simulink model "control_pos_6dof_conMI"  (R2023b)
settings: Solver=ode45  StartTime=0.0  StopTime=tsim  FixedStep=tstep  MaxStep=tstep
undefined symbols (not defined in the file): a0, a1, MI_Contr1, MI_Contr2, MI_Contr3, MI_Contr4, MI_Contr5, MI_Contr6, MI_motor1, MI_motor2, MI_motor3, MI_motor4, MI_motor5, MI_motor6, robot_params, sigbuilder_block, t_qeq_init, t_tr_init, tau_L, tr_ref
(part 2 of 10)

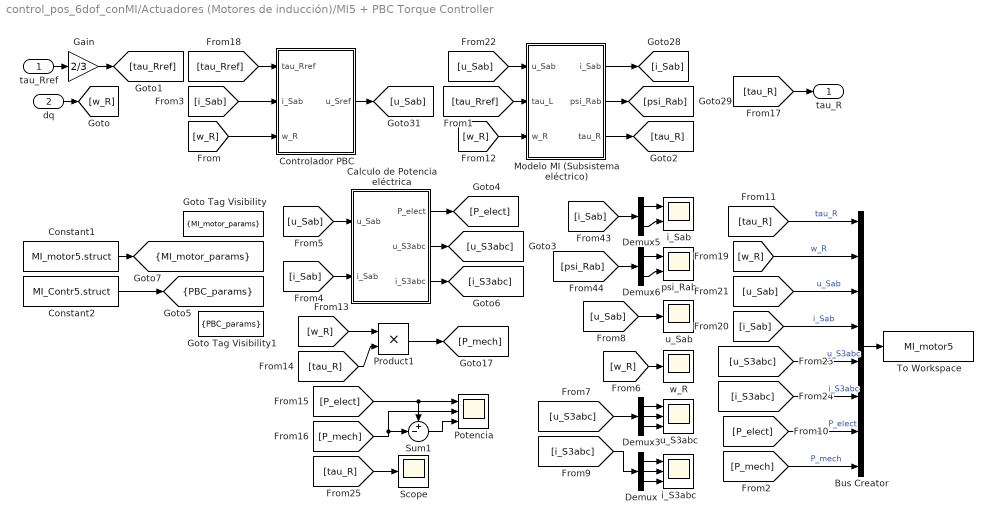
== system control_pos_6dof_conMI/Actuadores (Motores de inducción)/MI5 + PBC Torque Controller ==
  tau_Rref : Inport
  dq : Inport  Port=2
  Bus Creator : BusCreator  Inputs=8
  Calculo de Potencia eléctrica : Subsystem
  Constant1 : Constant  Value=MI_motor5.struct  OutDataTypeStr=Bus: MI_bus
  Constant2 : Constant  Value=MI_Contr5.struct  OutDataTypeStr=Bus: PBC_bus
  Controlador PBC : Subsystem
  Demux : Demux  Outputs=3
  Demux3 : Demux  Outputs=3
  Demux5 : Demux  Outputs=2
  Demux6 : Demux  Outputs=2
  Gain : Gain  Gain=2/3
  Goto Tag Visibility : GotoTagVisibility  GotoTag=MI_motor_params
  Goto Tag Visibility1 : GotoTagVisibility  GotoTag=PBC_params
  Modelo MI (Subsistema eléctrico) : Subsystem
  Potencia : Scope  NumInputPorts=3
  Product1 : Product
  Scope : Scope
  Sum1 : Sum  Inputs=+-|
  To Workspace : ToWorkspace  VariableName=MI_motor5  SaveFormat=Timeseries  SampleTime=-1
  i_S3abc : Scope  NumInputPorts=3
  i_Sab : Scope  NumInputPorts=2
  psi_Rab : Scope  NumInputPorts=2
  u_S3abc : Scope  NumInputPorts=3
  u_Sab : Scope
  w_R : Scope
  tau_R : Outport
  tag scope: MI_motor_params=scoped, PBC_params=scoped
  wires:
  Modelo MI (Subsistema eléctrico)/2(psi_Rab) -> [psi_Rab]
  [u_Sab] -> Modelo MI (Subsistema eléctrico)/1(u_Sab)
  [i_Sab] -> Controlador PBC/2(i_Sab)
  Controlador PBC/1(u_Sref) -> [u_Sab]
  [w_R] -> Controlador PBC/3(w_R)
  [tau_Rref] -> Modelo MI (Subsistema eléctrico)/2(tau_L)
  Calculo de Potencia eléctrica/2(u_S3abc) -> [u_S3abc]
  Calculo de Potencia eléctrica/1(P_elect) -> [P_elect]
  Demux5/1 -> i_Sab/1
  [w_R] -> w_R/1
  [u_Sab] -> Calculo de Potencia eléctrica/1(u_Sab)
  [psi_Rab] -> Demux6/1
  [u_Sab] -> u_Sab/1
  Demux6/1 -> psi_Rab/1
  Calculo de Potencia eléctrica/3(i_S3abc) -> [i_S3abc]
  Demux6/2 -> psi_Rab/2
  Demux5/2 -> i_Sab/2
  [i_Sab] -> Calculo de Potencia eléctrica/2(i_Sab)
  [i_Sab] -> Demux5/1
  Demux/2 -> i_S3abc/2
  Demux3/1 -> u_S3abc/1
  Demux3/3 -> u_S3abc/3
  [i_S3abc] -> Demux/1
  Demux/1 -> i_S3abc/1
  Demux/3 -> i_S3abc/3
  [u_S3abc] -> Demux3/1
  Demux3/2 -> u_S3abc/2
  Modelo MI (Subsistema eléctrico)/1(i_Sab) -> [i_Sab]
  Modelo MI (Subsistema eléctrico)/3(tau_R) -> [tau_R]
  Product1/1 -> [P_mech]
  [w_R] -> Product1/1
  [tau_R] -> Product1/2
  [tau_R] -> Bus Creator/1  "tau_R"
  Sum1/1 -> Potencia/3
  [P_elect] -> Potencia/1, Sum1/1
  [P_mech] -> Potencia/2, Sum1/2
  [tau_R] -> tau_R/1
  dq/1 -> [w_R]
  [tau_Rref] -> Controlador PBC/1(tau_Rref)
  [w_R] -> Modelo MI (Subsistema eléctrico)/3(w_R)
  Bus Creator/1 -> To Workspace/1
  Constant1/1 -> [MI_motor_params]
  [tau_R] -> Scope/1
  Constant2/1 -> [PBC_params]
  [w_R] -> Bus Creator/2  "w_R"
  [u_Sab] -> Bus Creator/3  "u_Sab"
  [i_Sab] -> Bus Creator/4  "i_Sab"
  [u_S3abc] -> Bus Creator/5  "u_S3abc"
  [i_S3abc] -> Bus Creator/6  "i_S3abc"
  [P_elect] -> Bus Creator/7  "P_elect"
  [P_mech] -> Bus Creator/8  "P_mech"
  Gain/1 -> [tau_Rref]
  tau_Rref/1 -> Gain/1

== system control_pos_6dof_conMI/Actuadores (Motores de inducción)/MI6 + PBC Torque Controller ==
  tau_Rref : Inport
  dq : Inport  Port=2
  Bus Creator : BusCreator  Inputs=8
  Calculo de Potencia eléctrica : Subsystem
  Constant1 : Constant  Value=MI_motor6.struct  OutDataTypeStr=Bus: MI_bus
  Constant2 : Constant  Value=MI_Contr6.struct  OutDataTypeStr=Bus: PBC_bus
  Controlador PBC : Subsystem
  Demux : Demux  Outputs=3
  Demux3 : Demux  Outputs=3
  Demux5 : Demux  Outputs=2
  Demux6 : Demux  Outputs=2
  Gain : Gain  Gain=2/3
  Goto Tag Visibility : GotoTagVisibility  GotoTag=MI_motor_params
  Goto Tag Visibility1 : GotoTagVisibility  GotoTag=PBC_params
  Modelo MI (Subsistema eléctrico) : Subsystem
  Potencia : Scope  NumInputPorts=3
  Product1 : Product
  Scope : Scope
  Sum1 : Sum  Inputs=+-|
  To Workspace : ToWorkspace  VariableName=MI_motor6  SaveFormat=Timeseries  SampleTime=-1
  i_S3abc : Scope  NumInputPorts=3
  i_Sab : Scope  NumInputPorts=2
  psi_Rab : Scope  NumInputPorts=2
  u_S3abc : Scope  NumInputPorts=3
  u_Sab : Scope
  w_R : Scope
  tau_R : Outport
  tag scope: MI_motor_params=scoped, PBC_params=scoped
  wires:
  Modelo MI (Subsistema eléctrico)/2(psi_Rab) -> [psi_Rab]
  [u_Sab] -> Modelo MI (Subsistema eléctrico)/1(u_Sab)
  [i_Sab] -> Controlador PBC/2(i_Sab)
  Controlador PBC/1(u_Sref) -> [u_Sab]
  [w_R] -> Controlador PBC/3(w_R)
  [tau_Rref] -> Modelo MI (Subsistema eléctrico)/2(tau_L)
  Calculo de Potencia eléctrica/2(u_S3abc) -> [u_S3abc]
  Calculo de Potencia eléctrica/1(P_elect) -> [P_elect]
  Demux5/1 -> i_Sab/1
  [w_R] -> w_R/1
  [u_Sab] -> Calculo de Potencia eléctrica/1(u_Sab)
  [psi_Rab] -> Demux6/1
  [u_Sab] -> u_Sab/1
  Demux6/1 -> psi_Rab/1
  Calculo de Potencia eléctrica/3(i_S3abc) -> [i_S3abc]
  Demux6/2 -> psi_Rab/2
  Demux5/2 -> i_Sab/2
  [i_Sab] -> Calculo de Potencia eléctrica/2(i_Sab)
  [i_Sab] -> Demux5/1
  Demux/2 -> i_S3abc/2
  Demux3/1 -> u_S3abc/1
  Demux3/3 -> u_S3abc/3
  [i_S3abc] -> Demux/1
  Demux/1 -> i_S3abc/1
  Demux/3 -> i_S3abc/3
  [u_S3abc] -> Demux3/1
  Demux3/2 -> u_S3abc/2
  Modelo MI (Subsistema eléctrico)/1(i_Sab) -> [i_Sab]
  Modelo MI (Subsistema eléctrico)/3(tau_R) -> [tau_R]
  Product1/1 -> [P_mech]
  [w_R] -> Product1/1
  [tau_R] -> Product1/2
  [tau_R] -> Bus Creator/1  "tau_R"
  Sum1/1 -> Potencia/3
  [P_elect] -> Potencia/1, Sum1/1
  [P_mech] -> Potencia/2, Sum1/2
  [tau_R] -> tau_R/1
  dq/1 -> [w_R]
  [tau_Rref] -> Controlador PBC/1(tau_Rref)
  [w_R] -> Modelo MI (Subsistema eléctrico)/3(w_R)
  Bus Creator/1 -> To Workspace/1
  Constant1/1 -> [MI_motor_params]
  [tau_R] -> Scope/1
  Constant2/1 -> [PBC_params]
  [w_R] -> Bus Creator/2  "w_R"
  [u_Sab] -> Bus Creator/3  "u_Sab"
  [i_Sab] -> Bus Creator/4  "i_Sab"
  [u_S3abc] -> Bus Creator/5  "u_S3abc"
  [i_S3abc] -> Bus Creator/6  "i_S3abc"
  [P_elect] -> Bus Creator/7  "P_elect"
  [P_mech] -> Bus Creator/8  "P_mech"
  Gain/1 -> [tau_Rref]
  tau_Rref/1 -> Gain/1

== system control_pos_6dof_conMI/Inicializar posición de robot manipulador/2 to 6 (3) ==
  In1 : Inport
  In2 : Inport  Port=2
  Demux4 : Demux  Outputs=6
  Demux6 : Demux  Outputs=6
  Mux{,1..5} (6 alike) : Mux  Inputs=2
  Out1 : Outport
  Out2 : Outport  Port=2
  Out3 : Outport  Port=3
  Out4 : Outport  Port=4
  Out5 : Outport  Port=5
  Out6 : Outport  Port=6
  wires:
  In2/1 -> Demux6/1
  Demux4/3 -> Mux2/1
  Demux4/5 -> Mux4/1
  Demux4/6 -> Mux5/1
  Demux6/5 -> Mux4/2
  Demux4/1 -> Mux/1
  Demux6/6 -> Mux5/2
  In1/1 -> Demux4/1
  Demux4/4 -> Mux3/1
  Demux6/2 -> Mux1/2
  Demux6/4 -> Mux3/2
  Demux6/1 -> Mux/2
  Demux4/2 -> Mux1/1
  Demux6/3 -> Mux2/2
  Mux/1 -> Out1/1
  Mux1/1 -> Out2/1
  Mux2/1 -> Out3/1
  Mux3/1 -> Out4/1
  Mux4/1 -> Out5/1
  Mux5/1 -> Out6/1

== system control_pos_6dof_conMI/Inicializar posición de robot manipulador/dq_init ==
  qfin : Inport
  t_fin : Inport  Port=2
  Demux : Demux  Outputs=6
  Mux : Mux  Inputs=6
  q1 : Subsystem
  q2 : Subsystem
  q3 : Subsystem
  q4 : Subsystem
  q5 : Subsystem
  q6 : Subsystem
  qpol : Outport
  wires:
  qfin/1 -> Demux/1
  t_fin/1 -> [t_fin]
  [t_fin] -> q1/2(t_fin)
  [t_fin] -> q2/2(t_fin)
  [t_fin] -> q3/2(t_fin)
  [t_fin] -> q4/2(t_fin)
  [t_fin] -> q5/2(t_fin)
  [t_fin] -> q6/2(t_fin)
  Mux/1 -> qpol/1
  Demux/1 -> q1/1(q_fin)
  Demux/2 -> q2/1(q_fin)
  Demux/3 -> q3/1(q_fin)
  Demux/4 -> q4/1(q_fin)
  Demux/5 -> q5/1(q_fin)
  Demux/6 -> q6/1(q_fin)
  q1/1(qpol) -> Mux/1
  q2/1(qpol) -> Mux/2
  q3/1(qpol) -> Mux/3
  q4/1(qpol) -> Mux/4
  q5/1(qpol) -> Mux/5
  q6/1(qpol) -> Mux/6

== system control_pos_6dof_conMI/Inicializar posición de robot manipulador/dq_init1 ==
  qfin : Inport
  t_fin : Inport  Port=2
  Demux : Demux  Outputs=6
  Mux : Mux  Inputs=6
  q1 : Subsystem
  q2 : Subsystem
  q3 : Subsystem
  q4 : Subsystem
  q5 : Subsystem
  q6 : Subsystem
  qpol : Outport
  wires:
  qfin/1 -> Demux/1
  t_fin/1 -> [t_fin]
  [t_fin] -> q1/2(t_fin)
  [t_fin] -> q2/2(t_fin)
  [t_fin] -> q3/2(t_fin)
  [t_fin] -> q4/2(t_fin)
  [t_fin] -> q5/2(t_fin)
  [t_fin] -> q6/2(t_fin)
  Mux/1 -> qpol/1
  Demux/1 -> q1/1(q_fin)
  Demux/2 -> q2/1(q_fin)
  Demux/3 -> q3/1(q_fin)
  Demux/4 -> q4/1(q_fin)
  Demux/5 -> q5/1(q_fin)
  Demux/6 -> q6/1(q_fin)
  q1/1(qpol) -> Mux/1
  q2/1(qpol) -> Mux/2
  q3/1(qpol) -> Mux/3
  q4/1(qpol) -> Mux/4
  q5/1(qpol) -> Mux/5
  q6/1(qpol) -> Mux/6

== system control_pos_6dof_conMI/Inicializar posición de robot manipulador/q_init ==
  q_eq : Inport
  q_init : Inport  Port=2
  t_init : Inport  Port=3
  t_fin : Inport  Port=4
  Clock : Clock
  Demux : Demux  Outputs=6
  Demux1 : Demux  Outputs=6
  Mux : Mux  Inputs=6
  Mux1 : Mux  Inputs=6
  Mux2 : Mux  Inputs=6
  init_q1 : Subsystem
  init_q2 : Subsystem
  init_q3 : Subsystem
  init_q4 : Subsystem
  init_q5 : Subsystem
  init_q6 : Subsystem
  q_fin : Outport
  dq_fin : Outport  Port=2
  ddq_fin : Outport  Port=3
  wires:
  t_fin/1 -> [tfin]
  [tfin] -> init_q1/5(t_fin)
  [tfin] -> init_q2/5(t_fin)
  [tfin] -> init_q3/5(t_fin)
  q_eq/1 -> Demux/1
  q_init/1 -> Demux1/1
  Demux/1 -> init_q1/2(q_eq)
  Demux/2 -> init_q2/2(q_eq)
  [t] -> init_q1/1(t)
  [t] -> init_q2/1(t)
  [t] -> init_q3/1(t)
  Demux/3 -> init_q3/2(q_eq)
  t_init/1 -> [t_init]
  [t_init] -> init_q1/4(t_init)
  [t_init] -> init_q2/4(t_init)
  [t_init] -> init_q3/4(t_init)
  Clock/1 -> [t]
  Demux1/1 -> init_q1/3(q_init)
  Demux1/2 -> init_q2/3(q_init)
  Demux1/3 -> init_q3/3(q_init)
  [t_init] -> init_q6/4(t_init)
  [t] -> init_q6/1(t)
  [tfin] -> init_q6/5(t_fin)
  [t_init] -> init_q4/4(t_init)
  [tfin] -> init_q4/5(t_fin)
  [t] -> init_q4/1(t)
  [t_init] -> init_q5/4(t_init)
  [tfin] -> init_q5/5(t_fin)
  [t] -> init_q5/1(t)
  Demux/4 -> init_q4/2(q_eq)
  Demux/5 -> init_q5/2(q_eq)
  Demux/6 -> init_q6/2(q_eq)
  Demux1/4 -> init_q4/3(q_init)
  Demux1/5 -> init_q5/3(q_init)
  Demux1/6 -> init_q6/3(q_init)
  init_q1/1(qpol) -> Mux/1
  init_q2/1(qpol) -> Mux/2
  init_q3/1(qpol) -> Mux/3
  init_q4/1(qpol) -> Mux/4
  init_q5/1(qpol) -> Mux/5
  init_q6/1(qpol) -> Mux/6
  init_q1/2(vpol) -> Mux1/1
  init_q2/2(vpol) -> Mux1/2
  init_q3/2(vpol) -> Mux1/3
  init_q4/2(vpol) -> Mux1/4
  init_q5/2(vpol) -> Mux1/5
  init_q6/2(vpol) -> Mux1/6
  init_q6/3(apol) -> Mux2/6
  init_q5/3(apol) -> Mux2/5
  init_q4/3(apol) -> Mux2/4
  init_q3/3(apol) -> Mux2/3
  init_q2/3(apol) -> Mux2/2
  init_q1/3(apol) -> Mux2/1
  Mux/1 -> q_fin/1
  Mux1/1 -> dq_fin/1
  Mux2/1 -> ddq_fin/1

== system control_pos_6dof_conMI/Inicializar posición de robot manipulador/q_init_tr ==
  q_init : Inport
  q_fin : Inport  Port=2
  t_fin : Inport  Port=3
  Demux : Demux  Outputs=6
  Demux1 : Demux  Outputs=6
  Mux : Mux  Inputs=6
  Mux1 : Mux  Inputs=6
  Mux2 : Mux  Inputs=6
  q1 : Subsystem
  q2 : Subsystem
  q3 : Subsystem
  q4 : Subsystem
  q5 : Subsystem
  q6 : Subsystem
  qpol : Outport
  vpol : Outport  Port=2
  apol : Outport  Port=3
  wires:
  q_fin/1 -> Demux/1
  t_fin/1 -> [t_fin]
  [t_fin] -> q1/3(t_fin)
  [t_fin] -> q2/3(t_fin)
  [t_fin] -> q3/3(t_fin)
  [t_fin] -> q4/3(t_fin)
  [t_fin] -> q5/3(t_fin)
  [t_fin] -> q6/3(t_fin)
  Mux/1 -> qpol/1
  Demux/1 -> q1/2(q_fin)
  Demux/2 -> q2/2(q_fin)
  Demux/3 -> q3/2(q_fin)
  Demux/4 -> q4/2(q_fin)
  Demux/5 -> q5/2(q_fin)
  Demux/6 -> q6/2(q_fin)
  q1/1(qpol) -> Mux/1
  q_init/1 -> Demux1/1
  Demux1/1 -> q1/1(q_init)
  Demux1/2 -> q2/1(q_init)
  Demux1/3 -> q3/1(q_init)
  Demux1/4 -> q4/1(q_init)
  Demux1/5 -> q5/1(q_init)
  Demux1/6 -> q6/1(q_init)
  q2/1(qpol) -> Mux/2
  q3/1(qpol) -> Mux/3
  q4/1(qpol) -> Mux/4
  q5/1(qpol) -> Mux/5
  q6/1(qpol) -> Mux/6
  Mux1/1 -> vpol/1
  Mux2/1 -> apol/1
  q1/2(vpol) -> Mux1/1
  q2/2(vpol) -> Mux1/2
  q3/2(vpol) -> Mux1/3
  q4/2(vpol) -> Mux1/4
  q5/2(vpol) -> Mux1/5
  q6/2(vpol) -> Mux1/6
  q1/3(apol) -> Mux2/1
  q2/3(apol) -> Mux2/2
  q3/3(apol) -> Mux2/3
  q4/3(apol) -> Mux2/4
  q5/3(apol) -> Mux2/5
  q6/3(apol) -> Mux2/6

== system control_pos_6dof_conMI/Actuadores (Motores de inducción)/MI1 + PBC Torque Controller/Calculo de Potencia eléctrica ==
  u_Sab : Inport
  i_Sab : Inport  Port=2
  Blondel-Park-i_Sab : MATLAB Function  TreatAsAtomicUnit=on
  Blondel-Park-u_Sab : MATLAB Function  TreatAsAtomicUnit=on
  Demux1 : Demux  Outputs=2
  Demux2 : Demux  Outputs=2
  Demux4 : Demux  Outputs=3
  Mux : Mux  Inputs=3
  Mux1 : Mux  Inputs=3
  Product1 : Product
  Sum1 : Sum  Inputs=|+++
  P_elect : Outport
  u_S3abc : Outport  Port=2
  i_S3abc : Outport  Port=3
  wires:
  Blondel-Park-u_Sab/2(U2) -> Mux1/2
  Blondel-Park-i_Sab/2(U2) -> Mux/2
  Blondel-Park-i_Sab/1(U1) -> Mux/1
  Blondel-Park-u_Sab/3(U3) -> Mux1/3
  Blondel-Park-i_Sab/3(U3) -> Mux/3
  Sum1/1 -> P_elect/1
  Demux2/2 -> Blondel-Park-u_Sab/2(BPU2)
  Demux2/1 -> Blondel-Park-u_Sab/1(BPU1)
  Demux1/2 -> Blondel-Park-i_Sab/2(BPU2)
  Demux4/1 -> Sum1/1
  [i_S3abc] -> Product1/2
  i_Sab/1 -> Demux2/1
  Blondel-Park-u_Sab/1(U1) -> Mux1/1
  Demux1/1 -> Blondel-Park-i_Sab/1(BPU1)
  Demux4/3 -> Sum1/3
  [u_S3abc] -> Product1/1
  Demux4/2 -> Sum1/2
  Product1/1 -> Demux4/1
  u_Sab/1 -> Demux1/1
  [u_S3abc] -> u_S3abc/1
  [i_S3abc] -> i_S3abc/1
  Mux/1 -> [u_S3abc]
  Mux1/1 -> [i_S3abc]

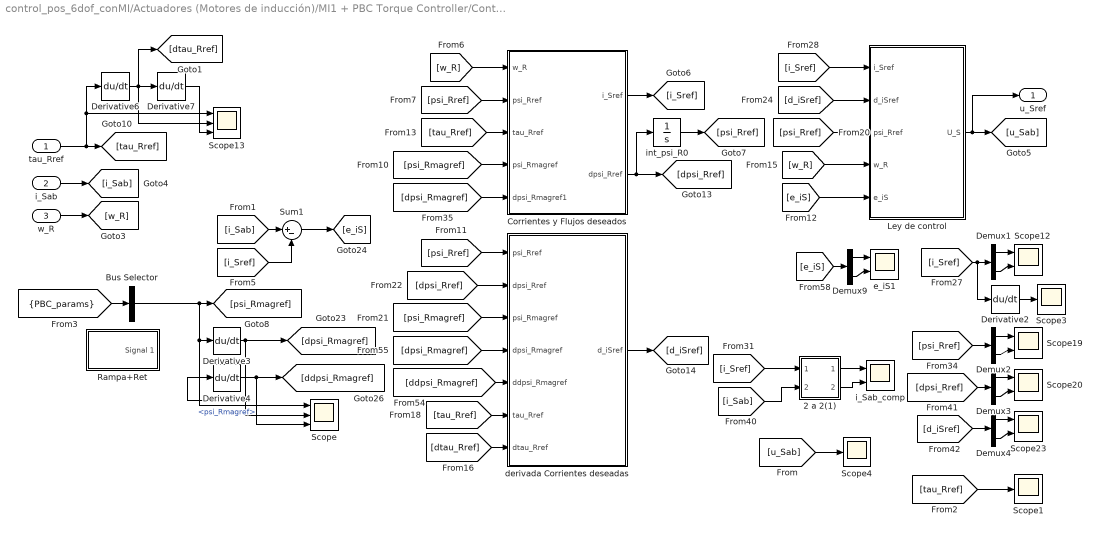
== system control_pos_6dof_conMI/Actuadores (Motores de inducción)/MI1 + PBC Torque Controller/Controlador PBC ==
  tau_Rref : Inport
  i_Sab : Inport  Port=2
  w_R : Inport  Port=3
  2 a 2(1) : Subsystem
  Bus Selector : BusSelector  OutputSignals=psi_Rmagref
  Corrientes y Flujos deseados : Subsystem
  Demux{1..4,9} (5 alike) : Demux  Outputs=2
  Derivative{2..4,6..7} (5 alike) : Derivative
  Ley de control : Subsystem
  Rampa+Ret : Subsystem  Tag=STV Subsys  LoadFcn=sigbuilder_block('load');  StartFcn=sigbuilder_block('start');  StopFcn=sigbuilder_block('stop');  ClipboardFcn=sigbuilder_block('clipboard');  mask(Sigbuilder block){tuvar=[0:10]}
      mask help: Sigbuilder GUI
      mask init:
      | if ~strcmp(get_param(bdroot(gcbh),'SimulationStatus'),'stopped') tuvar = sigbuilder_block('maskInit'); end
      settings: CopyFcn=sigbuilder_block('copy');  DeleteFcn=sigbuilder_block('delete');  ModelCloseFcn=sigbuilder_block('modelClose');  PreSaveFcn=sigbuilder_block('preSave');  PauseFcn=sigbuilder_block('pause')  ContinueFcn=sigbuilder_block('continue')  NameChangeFcn=sigbuilder_block('namechange');  OpenFcn=sigbuilder_block('open',[280.5 86.5 550.5 399.5 ]);  CloseFcn=sigbuilder_block('close');
      mask Display: plot(0, 0, 100, 100,[2, 2, 32, 32, 2], [68, 8, 8, 68, 68],[32, 2], [38, 38], [32, 19, 2],[53, 60, 44], [32, 17, 17, 2],[16, 16, 31, 31]);txt = getActiveGroup(gcbh);text(2, 100, txt,'verticalAlignment', 'top');
  Scope : Scope  NumInputPorts=3
  Scope1 : Scope
  Scope{12,19..20,23} (4 alike) : Scope  NumInputPorts=2
  Scope13 : Scope  NumInputPorts=3
  Scope3 : Scope
  Scope4 : Scope
  Sum1 : Sum  Inputs=|+-
  derivada Corrientes deseadas : Subsystem
  e_iS1 : Scope  NumInputPorts=2
  i_Sab_comp : Scope  NumInputPorts=2
  int_psi_R0 : Integrator  InitialCondition=[1.7041;0]
  u_Sref : Outport
  wires:
  Derivative3/1 -> Scope/2, Derivative4/1, [dpsi_Rmagref]
  Derivative4/1 -> [ddpsi_Rmagref], Scope/3
  Bus Selector/1 -> Scope/1, Derivative3/1, [psi_Rmagref]  "<psi_Rmagref>"
  i_Sab/1 -> [i_Sab]
  Demux1/1 -> Scope12/1
  [d_iSref] -> Demux4/1
  Demux3/2 -> Scope20/2
  Demux2/1 -> Scope19/1
  Demux1/2 -> Scope12/2
  [dpsi_Rref] -> Demux3/1
  Demux3/1 -> Scope20/1
  Demux4/1 -> Scope23/1
  [psi_Rref] -> Demux2/1
  Demux4/2 -> Scope23/2
  Demux2/2 -> Scope19/2
  [tau_Rref] -> Corrientes y Flujos deseados/3(tau_Rref)
  [w_R] -> Corrientes y Flujos deseados/1(w_R)
  int_psi_R0/1 -> [psi_Rref]
  Corrientes y Flujos deseados/2(dpsi_Rref) -> int_psi_R0/1, [dpsi_Rref]
  [psi_Rref] -> Corrientes y Flujos deseados/2(psi_Rref)
  [psi_Rmagref] -> Corrientes y Flujos deseados/4(psi_Rmagref)
  [dpsi_Rmagref] -> Corrientes y Flujos deseados/5(dpsi_Rmagref1)
  [psi_Rref] -> derivada Corrientes deseadas/1(psi_Rref)
  [dpsi_Rref] -> derivada Corrientes deseadas/2(dpsi_Rref)
  [psi_Rmagref] -> derivada Corrientes deseadas/3(psi_Rmagref)
  [dpsi_Rmagref] -> derivada Corrientes deseadas/4(dpsi_Rmagref)
  [ddpsi_Rmagref] -> derivada Corrientes deseadas/5(ddpsi_Rmagref)
  [tau_Rref] -> derivada Corrientes deseadas/6(tau_Rref)
  [dtau_Rref] -> derivada Corrientes deseadas/7(dtau_Rref)
  derivada Corrientes deseadas/1(d_iSref) -> [d_iSref]
  [e_iS] -> Demux9/1
  Demux9/1 -> e_iS1/1
  Demux9/2 -> e_iS1/2
  [i_Sab] -> Sum1/1
  [i_Sref] -> Sum1/2
  Sum1/1 -> [e_iS]
  [u_Sab] -> Scope4/1
  [i_Sref] -> Ley de control/1(i_Sref)
  [d_iSref] -> Ley de control/2(d_iSref)
  [psi_Rref] -> Ley de control/3(psi_Rref)
  [w_R] -> Ley de control/4(w_R)
  Ley de control/1(U_S) -> u_Sref/1, [u_Sab]
  [e_iS] -> Ley de control/5(e_iS)
  Derivative7/1 -> Scope13/3
  tau_Rref/1 -> Derivative6/1, Scope13/1, [tau_Rref]
  Derivative6/1 -> [dtau_Rref], Derivative7/1, Scope13/2
  2 a 2(1)/2(Out2) -> i_Sab_comp/2
  2 a 2(1)/1(Out1) -> i_Sab_comp/1
  [i_Sab] -> 2 a 2(1)/2(In2)
  [i_Sref] -> 2 a 2(1)/1(In1)
  [i_Sref] -> Derivative2/1, Demux1/1
  Derivative2/1 -> Scope3/1
  w_R/1 -> [w_R]
  [tau_Rref] -> Scope1/1
  [PBC_params] -> Bus Selector/1
  Corrientes y Flujos deseados/1(i_Sref) -> [i_Sref]

== system control_pos_6dof_conMI/Actuadores (Motores de inducción)/MI1 + PBC Torque Controller/Modelo MI (Subsistema eléctrico) ==
  u_Sab : Inport
  tau_L : Inport  Port=2
  w_R : Inport  Port=3
  Demux : Demux  Outputs=2
  Demux7 : Demux  Outputs=2
  Demux8 : Demux  Outputs=2
  Integrator : Integrator
  Integrator1 : Integrator
  Modelo Motor de inducción (Subsistema eléctrico) : MATLAB Function  TreatAsAtomicUnit=on
  Scope11 : Scope
  Scope3 : Scope  NumInputPorts=2
  Scope31 : Scope
  ab/dq : MATLAB Function  TreatAsAtomicUnit=on
  d_iSab : Scope  NumInputPorts=2
  dpsi_Rab1 : Scope  NumInputPorts=2
  i_Sab : Outport
  psi_Rab : Outport  Port=2
  tau_R : Outport  Port=3
  wires:
  Modelo Motor de inducción (Subsistema eléctrico)/1(di_Sab) -> Integrator/1, [d_iSab]
  Modelo Motor de inducción (Subsistema eléctrico)/2(dpsi_Rab) -> Integrator1/1, [dpsi_Rab]
  [w_R] -> Modelo Motor de inducción (Subsistema eléctrico)/5(w_R)
  [psi_Rab] -> Modelo Motor de inducción (Subsistema eléctrico)/4(psi_Rab)
  [i_Sab] -> Modelo Motor de inducción (Subsistema eléctrico)/3(i_Sab)
  Integrator1/1 -> [psi_Rab]
  u_Sab/1 -> [u_Sab]
  Modelo Motor de inducción (Subsistema eléctrico)/3(tau_R) -> [tau_R]
  [tau_R] -> Scope3/1
  ab/dq/1(psi_Rmag) -> Scope11/1
  [psi_Rab] -> Demux/1
  Demux7/1 -> dpsi_Rab1/1
  Demux7/2 -> dpsi_Rab1/2
  [d_iSab] -> Demux8/1
  ab/dq/2(rho) -> Scope31/1
  Demux/1 -> ab/dq/1(psi_ra)
  Demux8/2 -> d_iSab/2
  Demux8/1 -> d_iSab/1
  [dpsi_Rab] -> Demux7/1
  Demux/2 -> ab/dq/2(psi_rb)
  Integrator/1 -> [i_Sab]
  [MI_motor_params] -> Modelo Motor de inducción (Subsistema eléctrico)/1(MI_motor_params)
  [u_Sab] -> Modelo Motor de inducción (Subsistema eléctrico)/2(u_Sab)
  tau_L/1 -> [tau_L]
  [tau_L] -> Modelo Motor de inducción (Subsistema eléctrico)/6(tau_L)
  w_R/1 -> [w_R]
  [tau_R] -> tau_R/1
  [psi_Rab] -> psi_Rab/1
  [i_Sab] -> i_Sab/1
  [tau_L] -> Scope3/2

== system control_pos_6dof_conMI/Actuadores (Motores de inducción)/MI2 + PBC Torque Controller/Calculo de Potencia eléctrica ==
  u_Sab : Inport
  i_Sab : Inport  Port=2
  Blondel-Park-i_Sab : MATLAB Function  TreatAsAtomicUnit=on
  Blondel-Park-u_Sab : MATLAB Function  TreatAsAtomicUnit=on
  Demux1 : Demux  Outputs=2
  Demux2 : Demux  Outputs=2
  Demux4 : Demux  Outputs=3
  Mux : Mux  Inputs=3
  Mux1 : Mux  Inputs=3
  Product1 : Product
  Sum1 : Sum  Inputs=|+++
  P_elect : Outport
  u_S3abc : Outport  Port=2
  i_S3abc : Outport  Port=3
  wires:
  Blondel-Park-u_Sab/2(U2) -> Mux1/2
  Blondel-Park-i_Sab/2(U2) -> Mux/2
  Blondel-Park-i_Sab/1(U1) -> Mux/1
  Blondel-Park-u_Sab/3(U3) -> Mux1/3
  Blondel-Park-i_Sab/3(U3) -> Mux/3
  Sum1/1 -> P_elect/1
  Demux2/2 -> Blondel-Park-u_Sab/2(BPU2)
  Demux2/1 -> Blondel-Park-u_Sab/1(BPU1)
  Demux1/2 -> Blondel-Park-i_Sab/2(BPU2)
  Demux4/1 -> Sum1/1
  [i_S3abc] -> Product1/2
  i_Sab/1 -> Demux2/1
  Blondel-Park-u_Sab/1(U1) -> Mux1/1
  Demux1/1 -> Blondel-Park-i_Sab/1(BPU1)
  Demux4/3 -> Sum1/3
  [u_S3abc] -> Product1/1
  Demux4/2 -> Sum1/2
  Product1/1 -> Demux4/1
  u_Sab/1 -> Demux1/1
  [u_S3abc] -> u_S3abc/1
  [i_S3abc] -> i_S3abc/1
  Mux/1 -> [u_S3abc]
  Mux1/1 -> [i_S3abc]

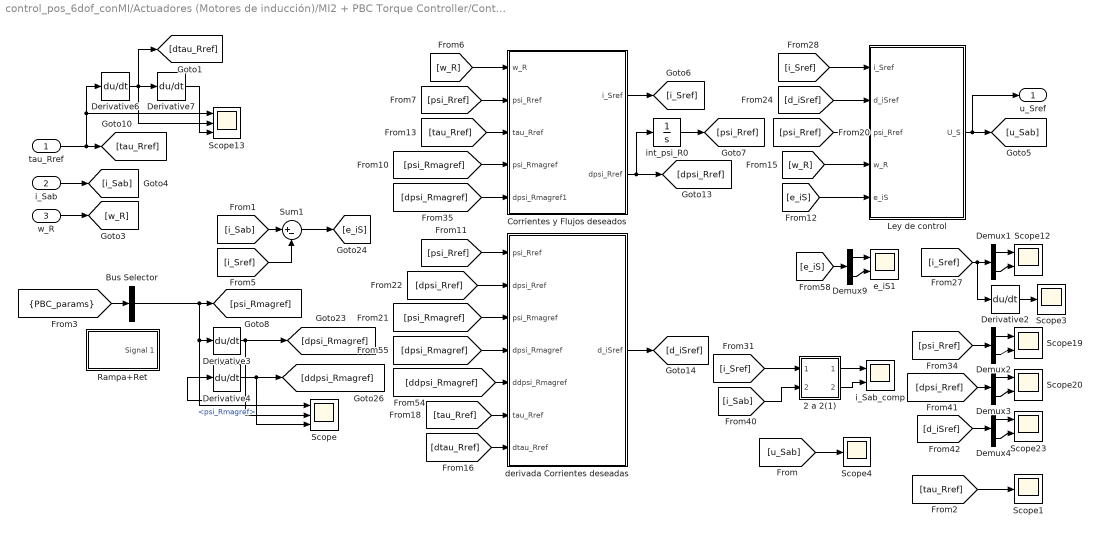
== system control_pos_6dof_conMI/Actuadores (Motores de inducción)/MI2 + PBC Torque Controller/Controlador PBC ==
  tau_Rref : Inport
  i_Sab : Inport  Port=2
  w_R : Inport  Port=3
  2 a 2(1) : Subsystem
  Bus Selector : BusSelector  OutputSignals=psi_Rmagref
  Corrientes y Flujos deseados : Subsystem
  Demux{1..4,9} (5 alike) : Demux  Outputs=2
  Derivative{2..4,6..7} (5 alike) : Derivative
  Ley de control : Subsystem
  Rampa+Ret : Subsystem  Tag=STV Subsys  LoadFcn=sigbuilder_block('load');  StartFcn=sigbuilder_block('start');  StopFcn=sigbuilder_block('stop');  ClipboardFcn=sigbuilder_block('clipboard');  mask(Sigbuilder block){tuvar=[0:10]}
      mask help: Sigbuilder GUI
      mask init:
      | if ~strcmp(get_param(bdroot(gcbh),'SimulationStatus'),'stopped') tuvar = sigbuilder_block('maskInit'); end
      settings: CopyFcn=sigbuilder_block('copy');  DeleteFcn=sigbuilder_block('delete');  ModelCloseFcn=sigbuilder_block('modelClose');  PreSaveFcn=sigbuilder_block('preSave');  PauseFcn=sigbuilder_block('pause')  ContinueFcn=sigbuilder_block('continue')  NameChangeFcn=sigbuilder_block('namechange');  OpenFcn=sigbuilder_block('open',[280.5 86.5 550.5 399.5 ]);  CloseFcn=sigbuilder_block('close');
      mask Display: plot(0, 0, 100, 100,[2, 2, 32, 32, 2], [68, 8, 8, 68, 68],[32, 2], [38, 38], [32, 19, 2],[53, 60, 44], [32, 17, 17, 2],[16, 16, 31, 31]);txt = getActiveGroup(gcbh);text(2, 100, txt,'verticalAlignment', 'top');
  Scope : Scope  NumInputPorts=3
  Scope1 : Scope
  Scope{12,19..20,23} (4 alike) : Scope  NumInputPorts=2
  Scope13 : Scope  NumInputPorts=3
  Scope3 : Scope
  Scope4 : Scope
  Sum1 : Sum  Inputs=|+-
  derivada Corrientes deseadas : Subsystem
  e_iS1 : Scope  NumInputPorts=2
  i_Sab_comp : Scope  NumInputPorts=2
  int_psi_R0 : Integrator  InitialCondition=[1.7456;0]
  u_Sref : Outport
  wires:
  Derivative3/1 -> Scope/2, Derivative4/1, [dpsi_Rmagref]
  Derivative4/1 -> [ddpsi_Rmagref], Scope/3
  Bus Selector/1 -> Scope/1, Derivative3/1, [psi_Rmagref]  "<psi_Rmagref>"
  i_Sab/1 -> [i_Sab]
  Demux1/1 -> Scope12/1
  [d_iSref] -> Demux4/1
  Demux3/2 -> Scope20/2
  Demux2/1 -> Scope19/1
  Demux1/2 -> Scope12/2
  [dpsi_Rref] -> Demux3/1
  Demux3/1 -> Scope20/1
  Demux4/1 -> Scope23/1
  [psi_Rref] -> Demux2/1
  Demux4/2 -> Scope23/2
  Demux2/2 -> Scope19/2
  [tau_Rref] -> Corrientes y Flujos deseados/3(tau_Rref)
  [w_R] -> Corrientes y Flujos deseados/1(w_R)
  int_psi_R0/1 -> [psi_Rref]
  Corrientes y Flujos deseados/2(dpsi_Rref) -> int_psi_R0/1, [dpsi_Rref]
  [psi_Rref] -> Corrientes y Flujos deseados/2(psi_Rref)
  [psi_Rmagref] -> Corrientes y Flujos deseados/4(psi_Rmagref)
  [dpsi_Rmagref] -> Corrientes y Flujos deseados/5(dpsi_Rmagref1)
  [psi_Rref] -> derivada Corrientes deseadas/1(psi_Rref)
  [dpsi_Rref] -> derivada Corrientes deseadas/2(dpsi_Rref)
  [psi_Rmagref] -> derivada Corrientes deseadas/3(psi_Rmagref)
  [dpsi_Rmagref] -> derivada Corrientes deseadas/4(dpsi_Rmagref)
  [ddpsi_Rmagref] -> derivada Corrientes deseadas/5(ddpsi_Rmagref)
  [tau_Rref] -> derivada Corrientes deseadas/6(tau_Rref)
  [dtau_Rref] -> derivada Corrientes deseadas/7(dtau_Rref)
  derivada Corrientes deseadas/1(d_iSref) -> [d_iSref]
  [e_iS] -> Demux9/1
  Demux9/1 -> e_iS1/1
  Demux9/2 -> e_iS1/2
  [i_Sab] -> Sum1/1
  [i_Sref] -> Sum1/2
  Sum1/1 -> [e_iS]
  [u_Sab] -> Scope4/1
  [i_Sref] -> Ley de control/1(i_Sref)
  [d_iSref] -> Ley de control/2(d_iSref)
  [psi_Rref] -> Ley de control/3(psi_Rref)
  [w_R] -> Ley de control/4(w_R)
  Ley de control/1(U_S) -> u_Sref/1, [u_Sab]
  [e_iS] -> Ley de control/5(e_iS)
  Derivative7/1 -> Scope13/3
  tau_Rref/1 -> Derivative6/1, Scope13/1, [tau_Rref]
  Derivative6/1 -> [dtau_Rref], Derivative7/1, Scope13/2
  2 a 2(1)/2(Out2) -> i_Sab_comp/2
  2 a 2(1)/1(Out1) -> i_Sab_comp/1
  [i_Sab] -> 2 a 2(1)/2(In2)
  [i_Sref] -> 2 a 2(1)/1(In1)
  [i_Sref] -> Derivative2/1, Demux1/1
  Derivative2/1 -> Scope3/1
  w_R/1 -> [w_R]
  [tau_Rref] -> Scope1/1
  [PBC_params] -> Bus Selector/1
  Corrientes y Flujos deseados/1(i_Sref) -> [i_Sref]

== system control_pos_6dof_conMI/Actuadores (Motores de inducción)/MI2 + PBC Torque Controller/Modelo MI (Subsistema eléctrico) ==
  u_Sab : Inport
  tau_L : Inport  Port=2
  w_R : Inport  Port=3
  Demux : Demux  Outputs=2
  Demux7 : Demux  Outputs=2
  Demux8 : Demux  Outputs=2
  Integrator : Integrator
  Integrator1 : Integrator
  Modelo Motor de inducción (Subsistema eléctrico) : MATLAB Function  TreatAsAtomicUnit=on
  Scope11 : Scope
  Scope3 : Scope  NumInputPorts=2
  Scope31 : Scope
  ab/dq : MATLAB Function  TreatAsAtomicUnit=on
  d_iSab : Scope  NumInputPorts=2
  dpsi_Rab1 : Scope  NumInputPorts=2
  i_Sab : Outport
  psi_Rab : Outport  Port=2
  tau_R : Outport  Port=3
  wires:
  Modelo Motor de inducción (Subsistema eléctrico)/1(di_Sab) -> Integrator/1, [d_iSab]
  Modelo Motor de inducción (Subsistema eléctrico)/2(dpsi_Rab) -> Integrator1/1, [dpsi_Rab]
  [w_R] -> Modelo Motor de inducción (Subsistema eléctrico)/5(w_R)
  [psi_Rab] -> Modelo Motor de inducción (Subsistema eléctrico)/4(psi_Rab)
  [i_Sab] -> Modelo Motor de inducción (Subsistema eléctrico)/3(i_Sab)
  Integrator1/1 -> [psi_Rab]
  u_Sab/1 -> [u_Sab]
  Modelo Motor de inducción (Subsistema eléctrico)/3(tau_R) -> [tau_R]
  [tau_R] -> Scope3/1
  ab/dq/1(psi_Rmag) -> Scope11/1
  [psi_Rab] -> Demux/1
  Demux7/1 -> dpsi_Rab1/1
  Demux7/2 -> dpsi_Rab1/2
  [d_iSab] -> Demux8/1
  ab/dq/2(rho) -> Scope31/1
  Demux/1 -> ab/dq/1(psi_ra)
  Demux8/2 -> d_iSab/2
  Demux8/1 -> d_iSab/1
  [dpsi_Rab] -> Demux7/1
  Demux/2 -> ab/dq/2(psi_rb)
  Integrator/1 -> [i_Sab]
  [MI_motor_params] -> Modelo Motor de inducción (Subsistema eléctrico)/1(MI_motor_params)
  [u_Sab] -> Modelo Motor de inducción (Subsistema eléctrico)/2(u_Sab)
  tau_L/1 -> [tau_L]
  [tau_L] -> Modelo Motor de inducción (Subsistema eléctrico)/6(tau_L)
  w_R/1 -> [w_R]
  [tau_R] -> tau_R/1
  [psi_Rab] -> psi_Rab/1
  [i_Sab] -> i_Sab/1
  [tau_L] -> Scope3/2

== system control_pos_6dof_conMI/Actuadores (Motores de inducción)/MI3 + PBC Torque Controller/Calculo de Potencia eléctrica ==
  u_Sab : Inport
  i_Sab : Inport  Port=2
  Blondel-Park-i_Sab : MATLAB Function  TreatAsAtomicUnit=on
  Blondel-Park-u_Sab : MATLAB Function  TreatAsAtomicUnit=on
  Demux1 : Demux  Outputs=2
  Demux2 : Demux  Outputs=2
  Demux4 : Demux  Outputs=3
  Mux : Mux  Inputs=3
  Mux1 : Mux  Inputs=3
  Product1 : Product
  Sum1 : Sum  Inputs=|+++
  P_elect : Outport
  u_S3abc : Outport  Port=2
  i_S3abc : Outport  Port=3
  wires:
  Blondel-Park-u_Sab/2(U2) -> Mux1/2
  Blondel-Park-i_Sab/2(U2) -> Mux/2
  Blondel-Park-i_Sab/1(U1) -> Mux/1
  Blondel-Park-u_Sab/3(U3) -> Mux1/3
  Blondel-Park-i_Sab/3(U3) -> Mux/3
  Sum1/1 -> P_elect/1
  Demux2/2 -> Blondel-Park-u_Sab/2(BPU2)
  Demux2/1 -> Blondel-Park-u_Sab/1(BPU1)
  Demux1/2 -> Blondel-Park-i_Sab/2(BPU2)
  Demux4/1 -> Sum1/1
  [i_S3abc] -> Product1/2
  i_Sab/1 -> Demux2/1
  Blondel-Park-u_Sab/1(U1) -> Mux1/1
  Demux1/1 -> Blondel-Park-i_Sab/1(BPU1)
  Demux4/3 -> Sum1/3
  [u_S3abc] -> Product1/1
  Demux4/2 -> Sum1/2
  Product1/1 -> Demux4/1
  u_Sab/1 -> Demux1/1
  [u_S3abc] -> u_S3abc/1
  [i_S3abc] -> i_S3abc/1
  Mux/1 -> [u_S3abc]
  Mux1/1 -> [i_S3abc]

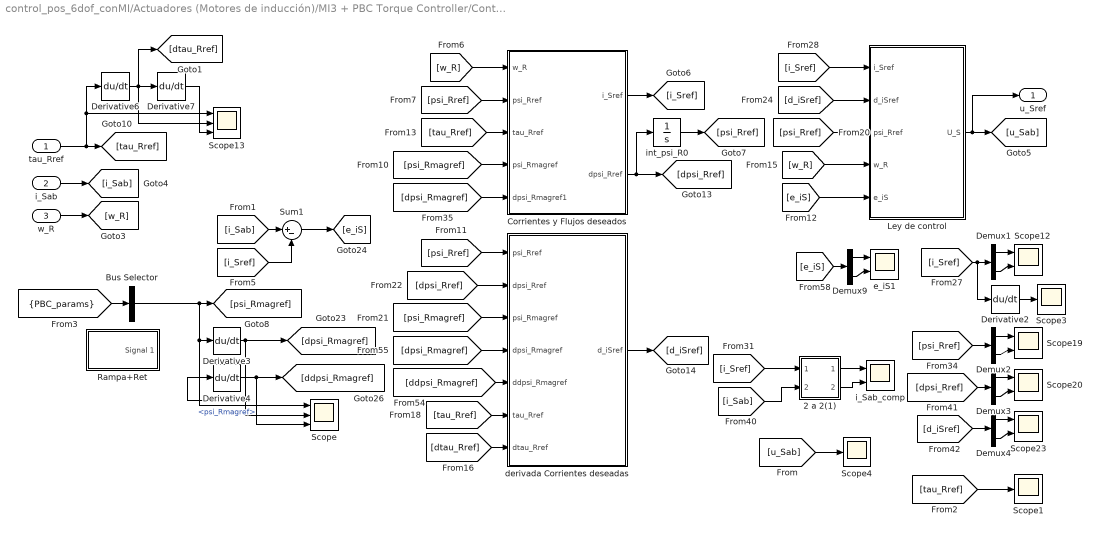
== system control_pos_6dof_conMI/Actuadores (Motores de inducción)/MI3 + PBC Torque Controller/Controlador PBC ==
  tau_Rref : Inport
  i_Sab : Inport  Port=2
  w_R : Inport  Port=3
  2 a 2(1) : Subsystem
  Bus Selector : BusSelector  OutputSignals=psi_Rmagref
  Corrientes y Flujos deseados : Subsystem
  Demux{1..4,9} (5 alike) : Demux  Outputs=2
  Derivative{2..4,6..7} (5 alike) : Derivative
  Ley de control : Subsystem
  Rampa+Ret : Subsystem  Tag=STV Subsys  LoadFcn=sigbuilder_block('load');  StartFcn=sigbuilder_block('start');  StopFcn=sigbuilder_block('stop');  ClipboardFcn=sigbuilder_block('clipboard');  mask(Sigbuilder block){tuvar=[0:10]}
      mask help: Sigbuilder GUI
      mask init:
      | if ~strcmp(get_param(bdroot(gcbh),'SimulationStatus'),'stopped') tuvar = sigbuilder_block('maskInit'); end
      settings: CopyFcn=sigbuilder_block('copy');  DeleteFcn=sigbuilder_block('delete');  ModelCloseFcn=sigbuilder_block('modelClose');  PreSaveFcn=sigbuilder_block('preSave');  PauseFcn=sigbuilder_block('pause')  ContinueFcn=sigbuilder_block('continue')  NameChangeFcn=sigbuilder_block('namechange');  OpenFcn=sigbuilder_block('open',[280.5 86.5 550.5 399.5 ]);  CloseFcn=sigbuilder_block('close');
      mask Display: plot(0, 0, 100, 100,[2, 2, 32, 32, 2], [68, 8, 8, 68, 68],[32, 2], [38, 38], [32, 19, 2],[53, 60, 44], [32, 17, 17, 2],[16, 16, 31, 31]);txt = getActiveGroup(gcbh);text(2, 100, txt,'verticalAlignment', 'top');
  Scope : Scope  NumInputPorts=3
  Scope1 : Scope
  Scope{12,19..20,23} (4 alike) : Scope  NumInputPorts=2
  Scope13 : Scope  NumInputPorts=3
  Scope3 : Scope
  Scope4 : Scope
  Sum1 : Sum  Inputs=|+-
  derivada Corrientes deseadas : Subsystem
  e_iS1 : Scope  NumInputPorts=2
  i_Sab_comp : Scope  NumInputPorts=2
  int_psi_R0 : Integrator  InitialCondition=[1.7041;0]
  u_Sref : Outport
  wires:
  Derivative3/1 -> Scope/2, Derivative4/1, [dpsi_Rmagref]
  Derivative4/1 -> [ddpsi_Rmagref], Scope/3
  Bus Selector/1 -> Scope/1, Derivative3/1, [psi_Rmagref]  "<psi_Rmagref>"
  i_Sab/1 -> [i_Sab]
  Demux1/1 -> Scope12/1
  [d_iSref] -> Demux4/1
  Demux3/2 -> Scope20/2
  Demux2/1 -> Scope19/1
  Demux1/2 -> Scope12/2
  [dpsi_Rref] -> Demux3/1
  Demux3/1 -> Scope20/1
  Demux4/1 -> Scope23/1
  [psi_Rref] -> Demux2/1
  Demux4/2 -> Scope23/2
  Demux2/2 -> Scope19/2
  [tau_Rref] -> Corrientes y Flujos deseados/3(tau_Rref)
  [w_R] -> Corrientes y Flujos deseados/1(w_R)
  int_psi_R0/1 -> [psi_Rref]
  Corrientes y Flujos deseados/2(dpsi_Rref) -> int_psi_R0/1, [dpsi_Rref]
  [psi_Rref] -> Corrientes y Flujos deseados/2(psi_Rref)
  [psi_Rmagref] -> Corrientes y Flujos deseados/4(psi_Rmagref)
  [dpsi_Rmagref] -> Corrientes y Flujos deseados/5(dpsi_Rmagref1)
  [psi_Rref] -> derivada Corrientes deseadas/1(psi_Rref)
  [dpsi_Rref] -> derivada Corrientes deseadas/2(dpsi_Rref)
  [psi_Rmagref] -> derivada Corrientes deseadas/3(psi_Rmagref)
  [dpsi_Rmagref] -> derivada Corrientes deseadas/4(dpsi_Rmagref)
  [ddpsi_Rmagref] -> derivada Corrientes deseadas/5(ddpsi_Rmagref)
  [tau_Rref] -> derivada Corrientes deseadas/6(tau_Rref)
  [dtau_Rref] -> derivada Corrientes deseadas/7(dtau_Rref)
  derivada Corrientes deseadas/1(d_iSref) -> [d_iSref]
  [e_iS] -> Demux9/1
  Demux9/1 -> e_iS1/1
  Demux9/2 -> e_iS1/2
  [i_Sab] -> Sum1/1
  [i_Sref] -> Sum1/2
  Sum1/1 -> [e_iS]
  [u_Sab] -> Scope4/1
  [i_Sref] -> Ley de control/1(i_Sref)
  [d_iSref] -> Ley de control/2(d_iSref)
  [psi_Rref] -> Ley de control/3(psi_Rref)
  [w_R] -> Ley de control/4(w_R)
  Ley de control/1(U_S) -> u_Sref/1, [u_Sab]
  [e_iS] -> Ley de control/5(e_iS)
  Derivative7/1 -> Scope13/3
  tau_Rref/1 -> Derivative6/1, Scope13/1, [tau_Rref]
  Derivative6/1 -> [dtau_Rref], Derivative7/1, Scope13/2
  2 a 2(1)/2(Out2) -> i_Sab_comp/2
  2 a 2(1)/1(Out1) -> i_Sab_comp/1
  [i_Sab] -> 2 a 2(1)/2(In2)
  [i_Sref] -> 2 a 2(1)/1(In1)
  [i_Sref] -> Derivative2/1, Demux1/1
  Derivative2/1 -> Scope3/1
  w_R/1 -> [w_R]
  [tau_Rref] -> Scope1/1
  [PBC_params] -> Bus Selector/1
  Corrientes y Flujos deseados/1(i_Sref) -> [i_Sref]

== system control_pos_6dof_conMI/Actuadores (Motores de inducción)/MI3 + PBC Torque Controller/Modelo MI (Subsistema eléctrico) ==
  u_Sab : Inport
  tau_L : Inport  Port=2
  w_R : Inport  Port=3
  Demux : Demux  Outputs=2
  Demux7 : Demux  Outputs=2
  Demux8 : Demux  Outputs=2
  Integrator : Integrator
  Integrator1 : Integrator
  Modelo Motor de inducción (Subsistema eléctrico) : MATLAB Function  TreatAsAtomicUnit=on
  Scope11 : Scope
  Scope3 : Scope  NumInputPorts=2
  Scope31 : Scope
  ab/dq : MATLAB Function  TreatAsAtomicUnit=on
  d_iSab : Scope  NumInputPorts=2
  dpsi_Rab1 : Scope  NumInputPorts=2
  i_Sab : Outport
  psi_Rab : Outport  Port=2
  tau_R : Outport  Port=3
  wires:
  Modelo Motor de inducción (Subsistema eléctrico)/1(di_Sab) -> Integrator/1, [d_iSab]
  Modelo Motor de inducción (Subsistema eléctrico)/2(dpsi_Rab) -> Integrator1/1, [dpsi_Rab]
  [w_R] -> Modelo Motor de inducción (Subsistema eléctrico)/5(w_R)
  [psi_Rab] -> Modelo Motor de inducción (Subsistema eléctrico)/4(psi_Rab)
  [i_Sab] -> Modelo Motor de inducción (Subsistema eléctrico)/3(i_Sab)
  Integrator1/1 -> [psi_Rab]
  u_Sab/1 -> [u_Sab]
  Modelo Motor de inducción (Subsistema eléctrico)/3(tau_R) -> [tau_R]
  [tau_R] -> Scope3/1
  ab/dq/1(psi_Rmag) -> Scope11/1
  [psi_Rab] -> Demux/1
  Demux7/1 -> dpsi_Rab1/1
  Demux7/2 -> dpsi_Rab1/2
  [d_iSab] -> Demux8/1
  ab/dq/2(rho) -> Scope31/1
  Demux/1 -> ab/dq/1(psi_ra)
  Demux8/2 -> d_iSab/2
  Demux8/1 -> d_iSab/1
  [dpsi_Rab] -> Demux7/1
  Demux/2 -> ab/dq/2(psi_rb)
  Integrator/1 -> [i_Sab]
  [MI_motor_params] -> Modelo Motor de inducción (Subsistema eléctrico)/1(MI_motor_params)
  [u_Sab] -> Modelo Motor de inducción (Subsistema eléctrico)/2(u_Sab)
  tau_L/1 -> [tau_L]
  [tau_L] -> Modelo Motor de inducción (Subsistema eléctrico)/6(tau_L)
  w_R/1 -> [w_R]
  [tau_R] -> tau_R/1
  [psi_Rab] -> psi_Rab/1
  [i_Sab] -> i_Sab/1
  [tau_L] -> Scope3/2

== system control_pos_6dof_conMI/Actuadores (Motores de inducción)/MI4 + PBC Torque Controller/Calculo de Potencia eléctrica ==
  u_Sab : Inport
  i_Sab : Inport  Port=2
  Blondel-Park-i_Sab : MATLAB Function  TreatAsAtomicUnit=on
  Blondel-Park-u_Sab : MATLAB Function  TreatAsAtomicUnit=on
  Demux1 : Demux  Outputs=2
  Demux2 : Demux  Outputs=2
  Demux4 : Demux  Outputs=3
  Mux : Mux  Inputs=3
  Mux1 : Mux  Inputs=3
  Product1 : Product
  Sum1 : Sum  Inputs=|+++
  P_elect : Outport
  u_S3abc : Outport  Port=2
  i_S3abc : Outport  Port=3
  wires:
  Blondel-Park-u_Sab/2(U2) -> Mux1/2
  Blondel-Park-i_Sab/2(U2) -> Mux/2
  Blondel-Park-i_Sab/1(U1) -> Mux/1
  Blondel-Park-u_Sab/3(U3) -> Mux1/3
  Blondel-Park-i_Sab/3(U3) -> Mux/3
  Sum1/1 -> P_elect/1
  Demux2/2 -> Blondel-Park-u_Sab/2(BPU2)
  Demux2/1 -> Blondel-Park-u_Sab/1(BPU1)
  Demux1/2 -> Blondel-Park-i_Sab/2(BPU2)
  Demux4/1 -> Sum1/1
  [i_S3abc] -> Product1/2
  i_Sab/1 -> Demux2/1
  Blondel-Park-u_Sab/1(U1) -> Mux1/1
  Demux1/1 -> Blondel-Park-i_Sab/1(BPU1)
  Demux4/3 -> Sum1/3
  [u_S3abc] -> Product1/1
  Demux4/2 -> Sum1/2
  Product1/1 -> Demux4/1
  u_Sab/1 -> Demux1/1
  [u_S3abc] -> u_S3abc/1
  [i_S3abc] -> i_S3abc/1
  Mux/1 -> [u_S3abc]
  Mux1/1 -> [i_S3abc]

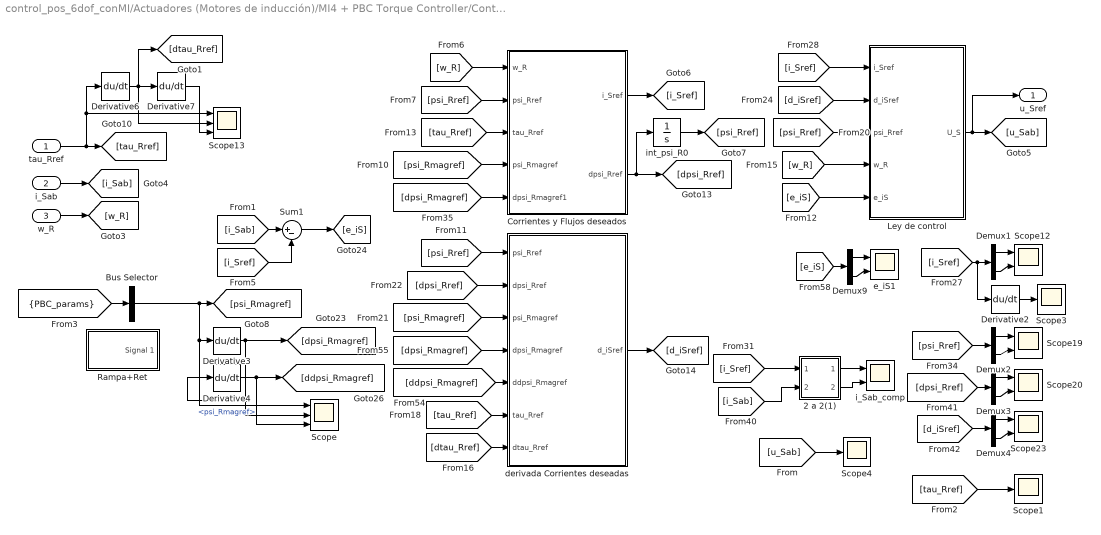
== system control_pos_6dof_conMI/Actuadores (Motores de inducción)/MI4 + PBC Torque Controller/Controlador PBC ==
  tau_Rref : Inport
  i_Sab : Inport  Port=2
  w_R : Inport  Port=3
  2 a 2(1) : Subsystem
  Bus Selector : BusSelector  OutputSignals=psi_Rmagref
  Corrientes y Flujos deseados : Subsystem
  Demux{1..4,9} (5 alike) : Demux  Outputs=2
  Derivative{2..4,6..7} (5 alike) : Derivative
  Ley de control : Subsystem
  Rampa+Ret : Subsystem  Tag=STV Subsys  LoadFcn=sigbuilder_block('load');  StartFcn=sigbuilder_block('start');  StopFcn=sigbuilder_block('stop');  ClipboardFcn=sigbuilder_block('clipboard');  mask(Sigbuilder block){tuvar=[0:10]}
      mask help: Sigbuilder GUI
      mask init:
      | if ~strcmp(get_param(bdroot(gcbh),'SimulationStatus'),'stopped') tuvar = sigbuilder_block('maskInit'); end
      settings: CopyFcn=sigbuilder_block('copy');  DeleteFcn=sigbuilder_block('delete');  ModelCloseFcn=sigbuilder_block('modelClose');  PreSaveFcn=sigbuilder_block('preSave');  PauseFcn=sigbuilder_block('pause')  ContinueFcn=sigbuilder_block('continue')  NameChangeFcn=sigbuilder_block('namechange');  OpenFcn=sigbuilder_block('open',[280.5 86.5 550.5 399.5 ]);  CloseFcn=sigbuilder_block('close');
      mask Display: plot(0, 0, 100, 100,[2, 2, 32, 32, 2], [68, 8, 8, 68, 68],[32, 2], [38, 38], [32, 19, 2],[53, 60, 44], [32, 17, 17, 2],[16, 16, 31, 31]);txt = getActiveGroup(gcbh);text(2, 100, txt,'verticalAlignment', 'top');
  Scope : Scope  NumInputPorts=3
  Scope1 : Scope
  Scope{12,19..20,23} (4 alike) : Scope  NumInputPorts=2
  Scope13 : Scope  NumInputPorts=3
  Scope3 : Scope
  Scope4 : Scope
  Sum1 : Sum  Inputs=|+-
  derivada Corrientes deseadas : Subsystem
  e_iS1 : Scope  NumInputPorts=2
  i_Sab_comp : Scope  NumInputPorts=2
  int_psi_R0 : Integrator  InitialCondition=[0.51032;0]
  u_Sref : Outport
  wires:
  Derivative3/1 -> Scope/2, Derivative4/1, [dpsi_Rmagref]
  Derivative4/1 -> [ddpsi_Rmagref], Scope/3
  Bus Selector/1 -> Scope/1, Derivative3/1, [psi_Rmagref]  "<psi_Rmagref>"
  i_Sab/1 -> [i_Sab]
  Demux1/1 -> Scope12/1
  [d_iSref] -> Demux4/1
  Demux3/2 -> Scope20/2
  Demux2/1 -> Scope19/1
  Demux1/2 -> Scope12/2
  [dpsi_Rref] -> Demux3/1
  Demux3/1 -> Scope20/1
  Demux4/1 -> Scope23/1
  [psi_Rref] -> Demux2/1
  Demux4/2 -> Scope23/2
  Demux2/2 -> Scope19/2
  [tau_Rref] -> Corrientes y Flujos deseados/3(tau_Rref)
  [w_R] -> Corrientes y Flujos deseados/1(w_R)
  int_psi_R0/1 -> [psi_Rref]
  Corrientes y Flujos deseados/2(dpsi_Rref) -> int_psi_R0/1, [dpsi_Rref]
  [psi_Rref] -> Corrientes y Flujos deseados/2(psi_Rref)
  [psi_Rmagref] -> Corrientes y Flujos deseados/4(psi_Rmagref)
  [dpsi_Rmagref] -> Corrientes y Flujos deseados/5(dpsi_Rmagref1)
  [psi_Rref] -> derivada Corrientes deseadas/1(psi_Rref)
  [dpsi_Rref] -> derivada Corrientes deseadas/2(dpsi_Rref)
  [psi_Rmagref] -> derivada Corrientes deseadas/3(psi_Rmagref)
  [dpsi_Rmagref] -> derivada Corrientes deseadas/4(dpsi_Rmagref)
  [ddpsi_Rmagref] -> derivada Corrientes deseadas/5(ddpsi_Rmagref)
  [tau_Rref] -> derivada Corrientes deseadas/6(tau_Rref)
  [dtau_Rref] -> derivada Corrientes deseadas/7(dtau_Rref)
  derivada Corrientes deseadas/1(d_iSref) -> [d_iSref]
  [e_iS] -> Demux9/1
  Demux9/1 -> e_iS1/1
  Demux9/2 -> e_iS1/2
  [i_Sab] -> Sum1/1
  [i_Sref] -> Sum1/2
  Sum1/1 -> [e_iS]
  [u_Sab] -> Scope4/1
  [i_Sref] -> Ley de control/1(i_Sref)
  [d_iSref] -> Ley de control/2(d_iSref)
  [psi_Rref] -> Ley de control/3(psi_Rref)
  [w_R] -> Ley de control/4(w_R)
  Ley de control/1(U_S) -> u_Sref/1, [u_Sab]
  [e_iS] -> Ley de control/5(e_iS)
  Derivative7/1 -> Scope13/3
  tau_Rref/1 -> Derivative6/1, Scope13/1, [tau_Rref]
  Derivative6/1 -> [dtau_Rref], Derivative7/1, Scope13/2
  2 a 2(1)/2(Out2) -> i_Sab_comp/2
  2 a 2(1)/1(Out1) -> i_Sab_comp/1
  [i_Sab] -> 2 a 2(1)/2(In2)
  [i_Sref] -> 2 a 2(1)/1(In1)
  [i_Sref] -> Derivative2/1, Demux1/1
  Derivative2/1 -> Scope3/1
  w_R/1 -> [w_R]
  [tau_Rref] -> Scope1/1
  [PBC_params] -> Bus Selector/1
  Corrientes y Flujos deseados/1(i_Sref) -> [i_Sref]

== system control_pos_6dof_conMI/Actuadores (Motores de inducción)/MI4 + PBC Torque Controller/Modelo MI (Subsistema eléctrico) ==
  u_Sab : Inport
  tau_L : Inport  Port=2
  w_R : Inport  Port=3
  Demux : Demux  Outputs=2
  Demux7 : Demux  Outputs=2
  Demux8 : Demux  Outputs=2
  Integrator : Integrator
  Integrator1 : Integrator
  Modelo Motor de inducción (Subsistema eléctrico) : MATLAB Function  TreatAsAtomicUnit=on
  Scope11 : Scope
  Scope3 : Scope  NumInputPorts=2
  Scope31 : Scope
  ab/dq : MATLAB Function  TreatAsAtomicUnit=on
  d_iSab : Scope  NumInputPorts=2
  dpsi_Rab1 : Scope  NumInputPorts=2
  i_Sab : Outport
  psi_Rab : Outport  Port=2
  tau_R : Outport  Port=3
  wires:
  Modelo Motor de inducción (Subsistema eléctrico)/1(di_Sab) -> Integrator/1, [d_iSab]
  Modelo Motor de inducción (Subsistema eléctrico)/2(dpsi_Rab) -> Integrator1/1, [dpsi_Rab]
  [w_R] -> Modelo Motor de inducción (Subsistema eléctrico)/5(w_R)
  [psi_Rab] -> Modelo Motor de inducción (Subsistema eléctrico)/4(psi_Rab)
  [i_Sab] -> Modelo Motor de inducción (Subsistema eléctrico)/3(i_Sab)
  Integrator1/1 -> [psi_Rab]
  u_Sab/1 -> [u_Sab]
  Modelo Motor de inducción (Subsistema eléctrico)/3(tau_R) -> [tau_R]
  [tau_R] -> Scope3/1
  ab/dq/1(psi_Rmag) -> Scope11/1
  [psi_Rab] -> Demux/1
  Demux7/1 -> dpsi_Rab1/1
  Demux7/2 -> dpsi_Rab1/2
  [d_iSab] -> Demux8/1
  ab/dq/2(rho) -> Scope31/1
  Demux/1 -> ab/dq/1(psi_ra)
  Demux8/2 -> d_iSab/2
  Demux8/1 -> d_iSab/1
  [dpsi_Rab] -> Demux7/1
  Demux/2 -> ab/dq/2(psi_rb)
  Integrator/1 -> [i_Sab]
  [MI_motor_params] -> Modelo Motor de inducción (Subsistema eléctrico)/1(MI_motor_params)
  [u_Sab] -> Modelo Motor de inducción (Subsistema eléctrico)/2(u_Sab)
  tau_L/1 -> [tau_L]
  [tau_L] -> Modelo Motor de inducción (Subsistema eléctrico)/6(tau_L)
  w_R/1 -> [w_R]
  [tau_R] -> tau_R/1
  [psi_Rab] -> psi_Rab/1
  [i_Sab] -> i_Sab/1
  [tau_L] -> Scope3/2

== system control_pos_6dof_conMI/Actuadores (Motores de inducción)/MI5 + PBC Torque Controller/Calculo de Potencia eléctrica ==
  u_Sab : Inport
  i_Sab : Inport  Port=2
  Blondel-Park-i_Sab : MATLAB Function  TreatAsAtomicUnit=on
  Blondel-Park-u_Sab : MATLAB Function  TreatAsAtomicUnit=on
  Demux1 : Demux  Outputs=2
  Demux2 : Demux  Outputs=2
  Demux4 : Demux  Outputs=3
  Mux : Mux  Inputs=3
  Mux1 : Mux  Inputs=3
  Product1 : Product
  Sum1 : Sum  Inputs=|+++
  P_elect : Outport
  u_S3abc : Outport  Port=2
  i_S3abc : Outport  Port=3
  wires:
  Blondel-Park-u_Sab/2(U2) -> Mux1/2
  Blondel-Park-i_Sab/2(U2) -> Mux/2
  Blondel-Park-i_Sab/1(U1) -> Mux/1
  Blondel-Park-u_Sab/3(U3) -> Mux1/3
  Blondel-Park-i_Sab/3(U3) -> Mux/3
  Sum1/1 -> P_elect/1
  Demux2/2 -> Blondel-Park-u_Sab/2(BPU2)
  Demux2/1 -> Blondel-Park-u_Sab/1(BPU1)
  Demux1/2 -> Blondel-Park-i_Sab/2(BPU2)
  Demux4/1 -> Sum1/1
  [i_S3abc] -> Product1/2
  i_Sab/1 -> Demux2/1
  Blondel-Park-u_Sab/1(U1) -> Mux1/1
  Demux1/1 -> Blondel-Park-i_Sab/1(BPU1)
  Demux4/3 -> Sum1/3
  [u_S3abc] -> Product1/1
  Demux4/2 -> Sum1/2
  Product1/1 -> Demux4/1
  u_Sab/1 -> Demux1/1
  [u_S3abc] -> u_S3abc/1
  [i_S3abc] -> i_S3abc/1
  Mux/1 -> [u_S3abc]
  Mux1/1 -> [i_S3abc]

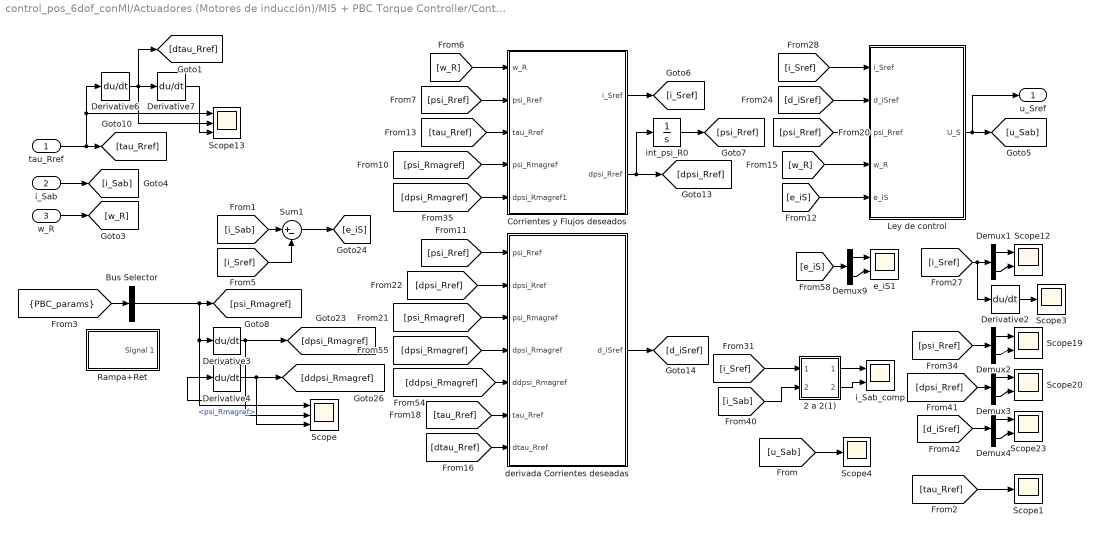
== system control_pos_6dof_conMI/Actuadores (Motores de inducción)/MI5 + PBC Torque Controller/Controlador PBC ==
  tau_Rref : Inport
  i_Sab : Inport  Port=2
  w_R : Inport  Port=3
  2 a 2(1) : Subsystem
  Bus Selector : BusSelector  OutputSignals=psi_Rmagref
  Corrientes y Flujos deseados : Subsystem
  Demux{1..4,9} (5 alike) : Demux  Outputs=2
  Derivative{2..4,6..7} (5 alike) : Derivative
  Ley de control : Subsystem
  Rampa+Ret : Subsystem  Tag=STV Subsys  LoadFcn=sigbuilder_block('load');  StartFcn=sigbuilder_block('start');  StopFcn=sigbuilder_block('stop');  ClipboardFcn=sigbuilder_block('clipboard');  mask(Sigbuilder block){tuvar=[0:10]}
      mask help: Sigbuilder GUI
      mask init:
      | if ~strcmp(get_param(bdroot(gcbh),'SimulationStatus'),'stopped') tuvar = sigbuilder_block('maskInit'); end
      settings: CopyFcn=sigbuilder_block('copy');  DeleteFcn=sigbuilder_block('delete');  ModelCloseFcn=sigbuilder_block('modelClose');  PreSaveFcn=sigbuilder_block('preSave');  PauseFcn=sigbuilder_block('pause')  ContinueFcn=sigbuilder_block('continue')  NameChangeFcn=sigbuilder_block('namechange');  OpenFcn=sigbuilder_block('open',[280.5 86.5 550.5 399.5 ]);  CloseFcn=sigbuilder_block('close');
      mask Display: plot(0, 0, 100, 100,[2, 2, 32, 32, 2], [68, 8, 8, 68, 68],[32, 2], [38, 38], [32, 19, 2],[53, 60, 44], [32, 17, 17, 2],[16, 16, 31, 31]);txt = getActiveGroup(gcbh);text(2, 100, txt,'verticalAlignment', 'top');
  Scope : Scope  NumInputPorts=3
  Scope1 : Scope
  Scope{12,19..20,23} (4 alike) : Scope  NumInputPorts=2
  Scope13 : Scope  NumInputPorts=3
  Scope3 : Scope
  Scope4 : Scope
  Sum1 : Sum  Inputs=|+-
  derivada Corrientes deseadas : Subsystem
  e_iS1 : Scope  NumInputPorts=2
  i_Sab_comp : Scope  NumInputPorts=2
  int_psi_R0 : Integrator  InitialCondition=[0.51032;0]
  u_Sref : Outport
  wires:
  Derivative3/1 -> Scope/2, Derivative4/1, [dpsi_Rmagref]
  Derivative4/1 -> [ddpsi_Rmagref], Scope/3
  Bus Selector/1 -> Scope/1, Derivative3/1, [psi_Rmagref]  "<psi_Rmagref>"
  i_Sab/1 -> [i_Sab]
  Demux1/1 -> Scope12/1
  [d_iSref] -> Demux4/1
  Demux3/2 -> Scope20/2
  Demux2/1 -> Scope19/1
  Demux1/2 -> Scope12/2
  [dpsi_Rref] -> Demux3/1
  Demux3/1 -> Scope20/1
  Demux4/1 -> Scope23/1
  [psi_Rref] -> Demux2/1
  Demux4/2 -> Scope23/2
  Demux2/2 -> Scope19/2
  [tau_Rref] -> Corrientes y Flujos deseados/3(tau_Rref)
  [w_R] -> Corrientes y Flujos deseados/1(w_R)
  int_psi_R0/1 -> [psi_Rref]
  Corrientes y Flujos deseados/2(dpsi_Rref) -> int_psi_R0/1, [dpsi_Rref]
  [psi_Rref] -> Corrientes y Flujos deseados/2(psi_Rref)
  [psi_Rmagref] -> Corrientes y Flujos deseados/4(psi_Rmagref)
  [dpsi_Rmagref] -> Corrientes y Flujos deseados/5(dpsi_Rmagref1)
  [psi_Rref] -> derivada Corrientes deseadas/1(psi_Rref)
  [dpsi_Rref] -> derivada Corrientes deseadas/2(dpsi_Rref)
  [psi_Rmagref] -> derivada Corrientes deseadas/3(psi_Rmagref)
  [dpsi_Rmagref] -> derivada Corrientes deseadas/4(dpsi_Rmagref)
  [ddpsi_Rmagref] -> derivada Corrientes deseadas/5(ddpsi_Rmagref)
  [tau_Rref] -> derivada Corrientes deseadas/6(tau_Rref)
  [dtau_Rref] -> derivada Corrientes deseadas/7(dtau_Rref)
  derivada Corrientes deseadas/1(d_iSref) -> [d_iSref]
  [e_iS] -> Demux9/1
  Demux9/1 -> e_iS1/1
  Demux9/2 -> e_iS1/2
  [i_Sab] -> Sum1/1
  [i_Sref] -> Sum1/2
  Sum1/1 -> [e_iS]
  [u_Sab] -> Scope4/1
  [i_Sref] -> Ley de control/1(i_Sref)
  [d_iSref] -> Ley de control/2(d_iSref)
  [psi_Rref] -> Ley de control/3(psi_Rref)
  [w_R] -> Ley de control/4(w_R)
  Ley de control/1(U_S) -> u_Sref/1, [u_Sab]
  [e_iS] -> Ley de control/5(e_iS)
  Derivative7/1 -> Scope13/3
  tau_Rref/1 -> Derivative6/1, Scope13/1, [tau_Rref]
  Derivative6/1 -> [dtau_Rref], Derivative7/1, Scope13/2
  2 a 2(1)/2(Out2) -> i_Sab_comp/2
  2 a 2(1)/1(Out1) -> i_Sab_comp/1
  [i_Sab] -> 2 a 2(1)/2(In2)
  [i_Sref] -> 2 a 2(1)/1(In1)
  [i_Sref] -> Derivative2/1, Demux1/1
  Derivative2/1 -> Scope3/1
  w_R/1 -> [w_R]
  [tau_Rref] -> Scope1/1
  [PBC_params] -> Bus Selector/1
  Corrientes y Flujos deseados/1(i_Sref) -> [i_Sref]

== system control_pos_6dof_conMI/Actuadores (Motores de inducción)/MI5 + PBC Torque Controller/Modelo MI (Subsistema eléctrico) ==
  u_Sab : Inport
  tau_L : Inport  Port=2
  w_R : Inport  Port=3
  Demux : Demux  Outputs=2
  Demux7 : Demux  Outputs=2
  Demux8 : Demux  Outputs=2
  Integrator : Integrator
  Integrator1 : Integrator
  Modelo Motor de inducción (Subsistema eléctrico) : MATLAB Function  TreatAsAtomicUnit=on
  Scope11 : Scope
  Scope3 : Scope  NumInputPorts=2
  Scope31 : Scope
  ab/dq : MATLAB Function  TreatAsAtomicUnit=on
  d_iSab : Scope  NumInputPorts=2
  dpsi_Rab1 : Scope  NumInputPorts=2
  i_Sab : Outport
  psi_Rab : Outport  Port=2
  tau_R : Outport  Port=3
  wires:
  Modelo Motor de inducción (Subsistema eléctrico)/1(di_Sab) -> Integrator/1, [d_iSab]
  Modelo Motor de inducción (Subsistema eléctrico)/2(dpsi_Rab) -> Integrator1/1, [dpsi_Rab]
  [w_R] -> Modelo Motor de inducción (Subsistema eléctrico)/5(w_R)
  [psi_Rab] -> Modelo Motor de inducción (Subsistema eléctrico)/4(psi_Rab)
  [i_Sab] -> Modelo Motor de inducción (Subsistema eléctrico)/3(i_Sab)
  Integrator1/1 -> [psi_Rab]
  u_Sab/1 -> [u_Sab]
  Modelo Motor de inducción (Subsistema eléctrico)/3(tau_R) -> [tau_R]
  [tau_R] -> Scope3/1
  ab/dq/1(psi_Rmag) -> Scope11/1
  [psi_Rab] -> Demux/1
  Demux7/1 -> dpsi_Rab1/1
  Demux7/2 -> dpsi_Rab1/2
  [d_iSab] -> Demux8/1
  ab/dq/2(rho) -> Scope31/1
  Demux/1 -> ab/dq/1(psi_ra)
  Demux8/2 -> d_iSab/2
  Demux8/1 -> d_iSab/1
  [dpsi_Rab] -> Demux7/1
  Demux/2 -> ab/dq/2(psi_rb)
  Integrator/1 -> [i_Sab]
  [MI_motor_params] -> Modelo Motor de inducción (Subsistema eléctrico)/1(MI_motor_params)
  [u_Sab] -> Modelo Motor de inducción (Subsistema eléctrico)/2(u_Sab)
  tau_L/1 -> [tau_L]
  [tau_L] -> Modelo Motor de inducción (Subsistema eléctrico)/6(tau_L)
  w_R/1 -> [w_R]
  [tau_R] -> tau_R/1
  [psi_Rab] -> psi_Rab/1
  [i_Sab] -> i_Sab/1
  [tau_L] -> Scope3/2

== system control_pos_6dof_conMI/Actuadores (Motores de inducción)/MI6 + PBC Torque Controller/Calculo de Potencia eléctrica ==
  u_Sab : Inport
  i_Sab : Inport  Port=2
  Blondel-Park-i_Sab : MATLAB Function  TreatAsAtomicUnit=on
  Blondel-Park-u_Sab : MATLAB Function  TreatAsAtomicUnit=on
  Demux1 : Demux  Outputs=2
  Demux2 : Demux  Outputs=2
  Demux4 : Demux  Outputs=3
  Mux : Mux  Inputs=3
  Mux1 : Mux  Inputs=3
  Product1 : Product
  Sum1 : Sum  Inputs=|+++
  P_elect : Outport
  u_S3abc : Outport  Port=2
  i_S3abc : Outport  Port=3
  wires:
  Blondel-Park-u_Sab/2(U2) -> Mux1/2
  Blondel-Park-i_Sab/2(U2) -> Mux/2
  Blondel-Park-i_Sab/1(U1) -> Mux/1
  Blondel-Park-u_Sab/3(U3) -> Mux1/3
  Blondel-Park-i_Sab/3(U3) -> Mux/3
  Sum1/1 -> P_elect/1
  Demux2/2 -> Blondel-Park-u_Sab/2(BPU2)
  Demux2/1 -> Blondel-Park-u_Sab/1(BPU1)
  Demux1/2 -> Blondel-Park-i_Sab/2(BPU2)
  Demux4/1 -> Sum1/1
  [i_S3abc] -> Product1/2
  i_Sab/1 -> Demux2/1
  Blondel-Park-u_Sab/1(U1) -> Mux1/1
  Demux1/1 -> Blondel-Park-i_Sab/1(BPU1)
  Demux4/3 -> Sum1/3
  [u_S3abc] -> Product1/1
  Demux4/2 -> Sum1/2
  Product1/1 -> Demux4/1
  u_Sab/1 -> Demux1/1
  [u_S3abc] -> u_S3abc/1
  [i_S3abc] -> i_S3abc/1
  Mux/1 -> [u_S3abc]
  Mux1/1 -> [i_S3abc]
